simulink library "INT_Brk_VD"  (R2016b)
settings: Solver=VariableStepAuto  StartTime=0.0  StopTime=10.0  RelTol=1e-3
settings Model: Creator=Administrator  LastModifiedBy=Administrator

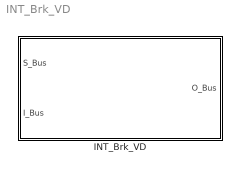
== system INT_Brk_VD ==
  INT_Brk_VD : Subsystem

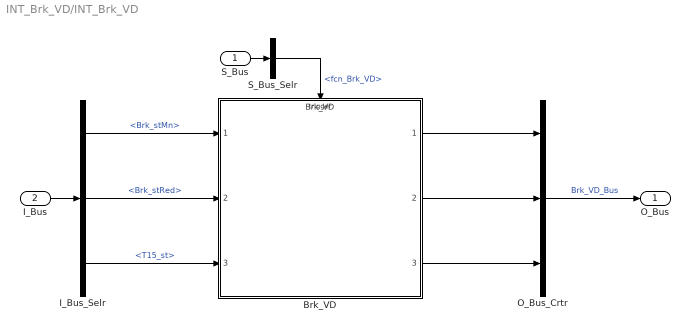
== system INT_Brk_VD/INT_Brk_VD ==
  S_Bus : Inport
  I_Bus : Inport  Port=2
  Brk_VD : ModelReference  ModelNameDialog=Brk_VD  SimulationMode=Normal  ModelReferenceVersion=1.10  TriggerPortName=function  TriggerPortTriggerType=function-call  TriggerPortStatesWhenEnabling=held
  I_Bus_Selr : BusSelector  OutputSignals=Brk_stMn,Brk_stRed,T15_st
  O_Bus_Crtr : BusCreator  Inputs=3
  S_Bus_Selr : BusSelector  OutputSignals=fcn_Brk_VD
  O_Bus : Outport
  wires:
  S_Bus_Selr/1 -> Brk_VD/Trigger  "<fcn_Brk_VD>"
  S_Bus/1 -> S_Bus_Selr/1
  I_Bus/1 -> I_Bus_Selr/1
  I_Bus_Selr/1 -> Brk_VD/1  "<Brk_stMn>"
  I_Bus_Selr/2 -> Brk_VD/2  "<Brk_stRed>"
  I_Bus_Selr/3 -> Brk_VD/3  "<T15_st>"
  O_Bus_Crtr/1 -> O_Bus/1  "Brk_VD_Bus"
  Brk_VD/1 -> O_Bus_Crtr/1
  Brk_VD/2 -> O_Bus_Crtr/2
  Brk_VD/3 -> O_Bus_Crtr/3
